simulink model "MotorPowerV1"  (R2023b)
settings: Solver=VariableStepAuto  StartTime=0.0  StopTime=100.899999999999  RelTol=1e-3
values from neighbouring files (symbols this model uses):
  airDensity = 1.293    [params.m]
  CdA = 0.3976    [params.m]
  g = 9.81    [params.m]
  radius = 0.65/2    (= 0.325)    [params.m]
  rollingResCoeff = 0.02    [params.m]
  totalMass = 310.5    [params.m]
settings Model: Creator=Sid Bagchi  LastModifiedBy=egeca
settings OptimizationCC: BlockReduction=off  DefaultParameterBehavior=Inlined  BufferReuse=off

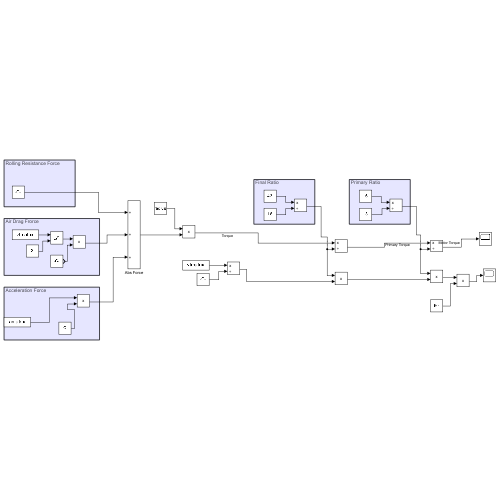
[thumbnail: Simulink's stored preview of the top-level diagram]
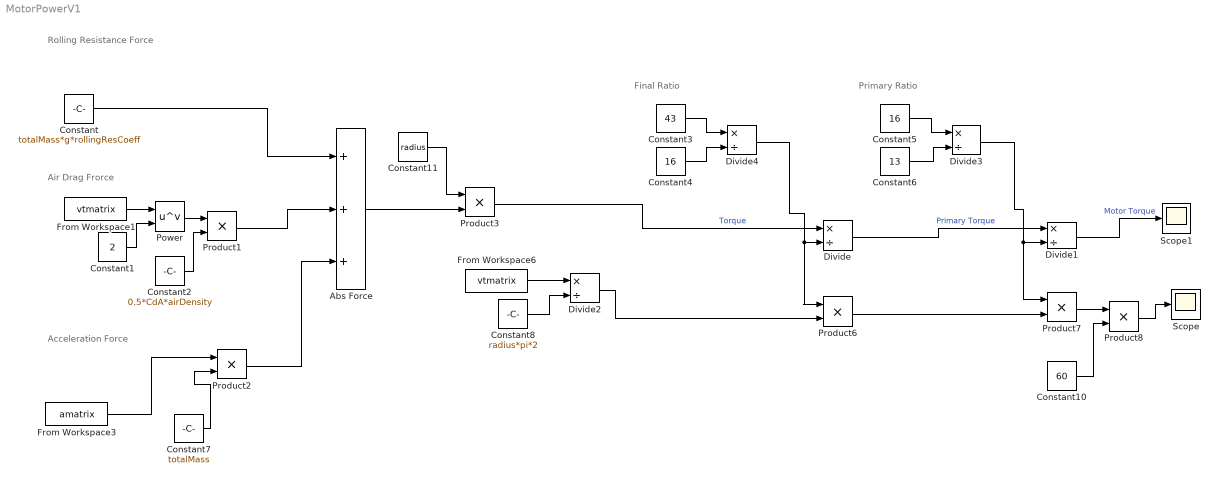
== system MotorPowerV1 ==
  note: Final Ratio
  note: Acceleration Force
  note: Air Drag Frorce
  note: Rolling Resistance Force
  note: Primary Ratio
  Abs Force : Sum  Inputs=+++
  Constant : Constant  Value=totalMass*g*rollingResCoeff
  Constant1 : Constant  Value=2
  Constant10 : Constant  Value=60
  Constant11 : Constant  Value=radius
  Constant2 : Constant  Value=0.5*CdA*airDensity
  Constant3 : Constant  Value=43
  Constant4 : Constant  Value=16
  Constant5 : Constant  Value=16
  Constant6 : Constant  Value=13
  Constant7 : Constant  Value=totalMass
  Constant8 : Constant  Value=radius*pi*2
  Divide{,1..4} (5 alike) : Product  Inputs=*/
  From Workspace1 : FromWorkspace  VariableName=vtmatrix
  From Workspace3 : FromWorkspace  VariableName=amatrix
  From Workspace6 : FromWorkspace  VariableName=vtmatrix
  Power : Math  Operator=pow
  Product{1..3,6..8} (6 alike) : Product
  Scope : Scope
  Scope1 : Scope
  wires:
  Constant/1 -> Abs Force/1
  Constant1/1 -> Power/2
  From Workspace1/1 -> Power/1
  Power/1 -> Product1/1
  Product1/1 -> Abs Force/2
  Constant2/1 -> Product1/2
  Constant7/1 -> Product2/2
  From Workspace3/1 -> Product2/1
  Product2/1 -> Abs Force/3
  Abs Force/1 -> Product3/2
  From Workspace6/1 -> Divide2/1
  Constant8/1 -> Divide2/2
  Divide2/1 -> Product6/2
  Constant3/1 -> Divide4/1
  Constant4/1 -> Divide4/2
  Divide/1 -> Divide1/1  "Primary Torque"
  Constant6/1 -> Divide3/2
  Constant5/1 -> Divide3/1
  Divide1/1 -> Scope1/1  "Motor Torque"
  Product6/1 -> Product7/2
  Product7/1 -> Product8/1
  Product8/1 -> Scope/1
  Constant10/1 -> Product8/2
  Constant11/1 -> Product3/1
  Product3/1 -> Divide/1  "Torque"
  Divide4/1 -> Product6/1, Divide/2
  Divide3/1 -> Product7/1, Divide1/2
